simulink model "RIP1"  (R2015a)
settings: Solver=ode45  StartTime=0.0  StopTime=30  RelTol=1e-6
values from neighbouring files (symbols this model uses):
  d0 = 1.5897e-3    (= 0.0015897)    [initialise.m]
  d1 = 1.773e-6    (= 1.773e-06)    [initialise.m]
  g = 9.81    [initialise.m]
  J0 = 1.4316e-4    (= 0.00014316)    [initialise.m]
  J1 = 2.078867e-4    (= 0.0002078867)    [initialise.m]
  Kf = 0.05722    [initialise.m]
  Kg = 13/18    (= 0.722222222222)    [initialise.m]
  Kt = 0.05722    [initialise.m]
  L0 = 0.09    [initialise.m]
  L1 = 0.225    [initialise.m]
  m1 = 0.009    [initialise.m]
  Ra = 17    [initialise.m]
settings Model: Creator=Alvin  LastModifiedBy=Alvin
settings SolverCC: AlgebraicLoopSolver=LineSearch
settings DataIOCC: SaveState=on

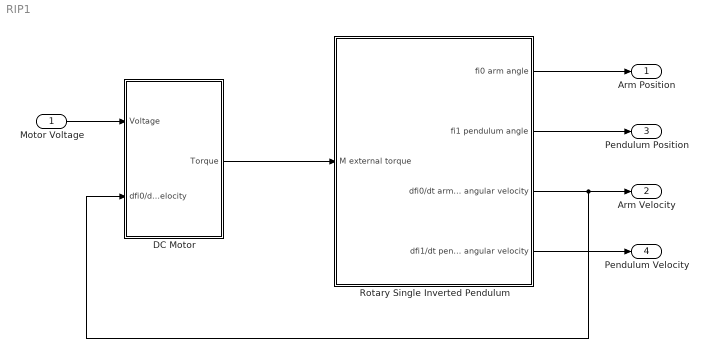
== system RIP1 ==
  Motor Voltage : Inport
  DC Motor : Subsystem
  Rotary Single Inverted Pendulum : Subsystem
  Arm Position : Outport
  Arm Velocity : Outport  Port=2
  Pendulum Position : Outport  Port=3
  Pendulum Velocity : Outport  Port=4
  wires:
  DC Motor/1(Torque) -> Rotary Single Inverted Pendulum/1(M external torque)
  Rotary Single Inverted Pendulum/3(dfi0/dt arm angular velocity) -> Arm Velocity/1, DC Motor/2(dfi0/dt Arm Angular Velocity)
  Motor Voltage/1 -> DC Motor/1(Voltage)
  Rotary Single Inverted Pendulum/1(fi0 arm angle) -> Arm Position/1
  Rotary Single Inverted Pendulum/2(fi1 pendulum angle) -> Pendulum Position/1
  Rotary Single Inverted Pendulum/4(dfi1/dt pendulum angular velocity) -> Pendulum Velocity/1

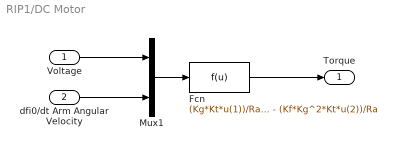
== system RIP1/DC Motor ==
  Voltage : Inport
  dfi0/dt Arm Angular Velocity : Inport  Port=2
  Fcn : Fcn  Expr=(Kg*Kt*u(1))/Ra - (Kf*Kg^2*Kt*u(2))/Ra
  Mux1 : Mux  Inputs=2
  Torque : Outport
  wires:
  dfi0/dt Arm Angular Velocity/1 -> Mux1/2
  Voltage/1 -> Mux1/1
  Mux1/1 -> Fcn/1
  Fcn/1 -> Torque/1

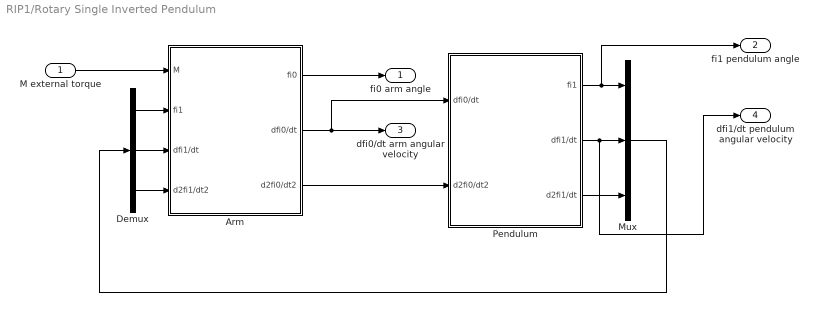
== system RIP1/Rotary Single Inverted Pendulum ==
  M external torque : Inport
  Arm : Subsystem
  Demux : Demux  Outputs=3
  Mux : Mux  Inputs=3
  Pendulum : Subsystem
  fi0 arm angle : Outport
  fi1 pendulum angle : Outport  Port=2
  dfi0/dt arm angular velocity : Outport  Port=3
  dfi1/dt pendulum angular velocity : Outport  Port=4
  wires:
  Pendulum/1(fi1) -> fi1 pendulum angle/1, Mux/1
  Pendulum/2(dfi1/dt) -> dfi1/dt pendulum angular velocity/1, Mux/2
  Mux/1 -> Demux/1
  Demux/1 -> Arm/2(fi1)
  Demux/2 -> Arm/3(dfi1/dt)
  Demux/3 -> Arm/4(d2fi1/dt2)
  M external torque/1 -> Arm/1(M)
  Pendulum/3(d2fi1/dt) -> Mux/3
  Arm/3(d2fi0/dt2) -> Pendulum/2(d2fi0/dt2)
  Arm/1(fi0) -> fi0 arm angle/1
  Arm/2(dfi0/dt) -> dfi0/dt arm angular velocity/1, Pendulum/1(dfi0/dt)

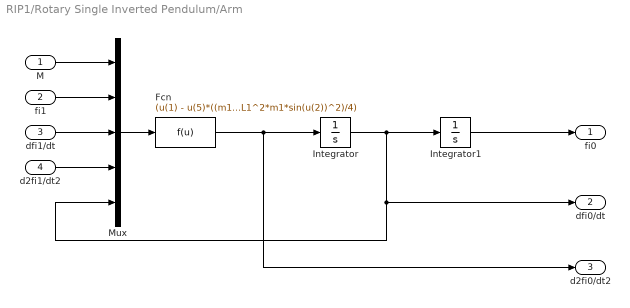
== system RIP1/Rotary Single Inverted Pendulum/Arm ==
  M : Inport
  fi1 : Inport  Port=2
  dfi1/dt : Inport  Port=3
  d2fi1/dt2 : Inport  Port=4
  Fcn : Fcn  Expr=(u(1) - u(5)*((m1*u(3)*sin(2*u(2))*L1^2)/4 + d0) + (L0*L1*m1*u(3)^2*sin(u(2)))/2 - (L0*L1*m1*u(4)*cos(u(2)))/2)/(J0 + L0^2*m1 + (L1^2*m1*sin(u(2))^2)/4)
  Integrator : Integrator
  Integrator1 : Integrator
  Mux : Mux  Inputs=5
  fi0 : Outport
  dfi0/dt : Outport  Port=2
  d2fi0/dt2 : Outport  Port=3
  wires:
  Mux/1 -> Fcn/1
  Fcn/1 -> d2fi0/dt2/1, Integrator/1
  Integrator/1 -> dfi0/dt/1, Mux/5, Integrator1/1
  Integrator1/1 -> fi0/1
  fi1/1 -> Mux/2
  dfi1/dt/1 -> Mux/3
  M/1 -> Mux/1
  d2fi1/dt2/1 -> Mux/4

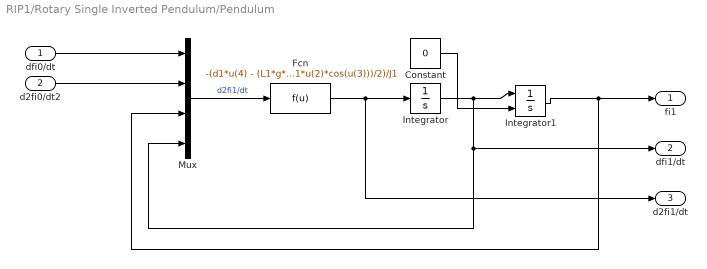
== system RIP1/Rotary Single Inverted Pendulum/Pendulum ==
  dfi0/dt : Inport
  d2fi0/dt2 : Inport  Port=2
  Constant : Constant  Value=0
  Fcn : Fcn  Expr=-(d1*u(4) - (L1*g*m1*sin(u(3)))/2 - (L1^2*m1*u(1)^2*sin(2*u(3)))/8 + (L0*L1*m1*u(2)*cos(u(3)))/2)/J1
  Integrator : Integrator
  Integrator1 : Integrator  InitialConditionSource=external
  Mux : Mux
  fi1 : Outport
  dfi1/dt : Outport  Port=2
  d2fi1/dt : Outport  Port=3
  wires:
  Integrator1/1 -> fi1/1, Mux/3
  Fcn/1 -> d2fi1/dt/1, Integrator/1
  Mux/1 -> Fcn/1  "d2fi1/dt"
  Integrator/1 -> dfi1/dt/1, Mux/4, Integrator1/1
  dfi0/dt/1 -> Mux/1
  d2fi0/dt2/1 -> Mux/2
  Constant/1 -> Integrator1/2
